simulink model "UDPsimulink"  (R2021a)
settings: Solver=VariableStepAuto  StartTime=0.0  StopTime=inf  RelTol=1e-3
libraries: hostiolib x1, instrumentlib x1
settings Model: EnablePacing=on  Creator=sanja  LastModifiedBy=sanja

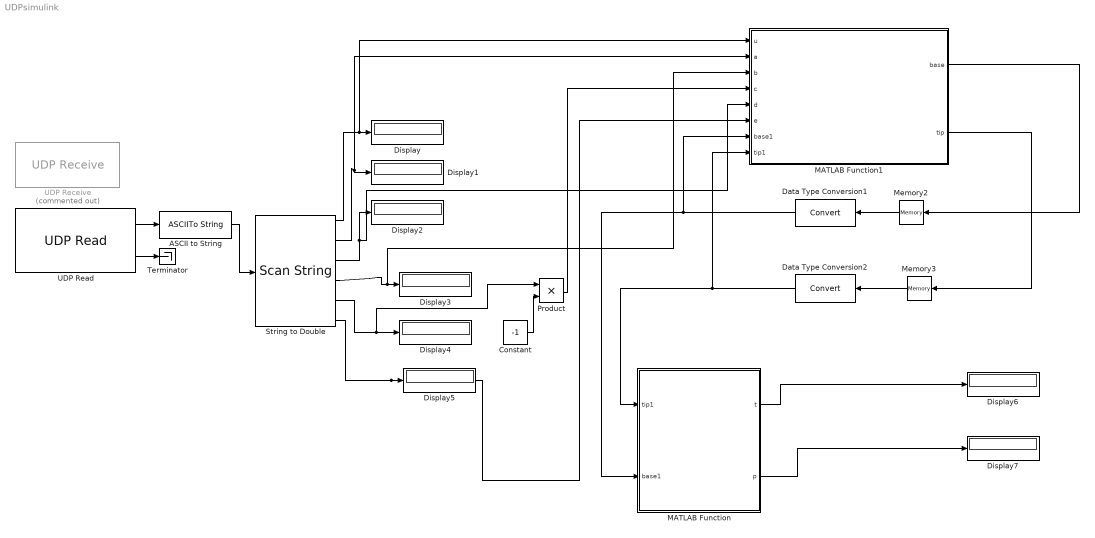
== system UDPsimulink ==
  ASCII to String : ASCIIToString
  Constant : Constant  Value=-1
  Data Type Conversion1 : DataTypeConversion
  Data Type Conversion2 : DataTypeConversion
  Display{,1..7} (8 alike) : Display
  MATLAB Function : MATLAB Function  TreatAsAtomicUnit=on
  MATLAB Function1 : MATLAB Function  TreatAsAtomicUnit=on
  Memory2 : Memory  InitialCondition=[0.0,0,0,0,0,1]  InheritSampleTime=on
  Memory3 : Memory  InitialCondition=[1.0,0,0,0,0,1]  InheritSampleTime=on
  Product : Product
  String to Double : ScanString  Format="\"%f %f %f %f %f %f\""
  Terminator : Terminator
  UDP Read : hostiolib/UDP Read  localURL='0.0.0.0'  localPort=60002  remoteURL='localhost'  remotePort=-1  recvBufferSize=1024  dims=255  signalDatatype=uint8  isVarSize=off  showBlockingTime=on  blockingTime=0  sampletime=0.001  blockPlatform=HOST  hoistedMaskSrc=UDP Read/UDP Read Sim/UDP Read
      settings: SourceProductBaseCode=HW
  UDP Receive : instrumentlib/UDP Receive  Commented=on  Host=localhost  Port=60001  LocalPort=60002  EnablePortSharing=off  GetLatestData=off  DataSize="[1  9]"  DataType=uint8  ASCIIFormatting=%f %f  Terminator=127  ByteOrder=BigEndian  EnableBlockingMode=on  Timeout=10  SampleTime=0.01  LocalAddress=localhost
  wires:
  ASCII to String/1 -> String to Double/1
  String to Double/1 -> MATLAB Function1/1(u), Display/1
  UDP Read/2 -> Terminator/1
  UDP Read/1 -> ASCII to String/1
  String to Double/3 -> MATLAB Function1/5(d), Display2/1
  String to Double/5 -> Product/1, Display4/1
  String to Double/6 -> MATLAB Function1/6(e), Display5/1
  String to Double/2 -> Display1/1, MATLAB Function1/2(a)
  String to Double/4 -> MATLAB Function1/3(b), Display3/1
  MATLAB Function/1(t) -> Display6/1
  MATLAB Function/2(p) -> Display7/1
  Memory2/1 -> Data Type Conversion1/1
  MATLAB Function1/1(base) -> Memory2/1
  Data Type Conversion1/1 -> MATLAB Function/2(base1), MATLAB Function1/7(base1)
  Memory3/1 -> Data Type Conversion2/1
  MATLAB Function1/2(tip) -> Memory3/1
  Data Type Conversion2/1 -> MATLAB Function/1(tip1), MATLAB Function1/8(tip1)
  Constant/1 -> Product/2
  Product/1 -> MATLAB Function1/4(c)

== matlab function UDPsimulink/MATLAB Function1 ==
  data: u input; base output; a input; b input; c input; d input; e input; base1 input; tip1 input; tip output
function [base,tip]= fcn(u,a,b,c,d,e,base1,tip1)
if u==0.0
    %base1=[double(u),double(a),double(b),double(c),double(d),double(e)];
    base1(1)=double(u);
    base1(2)=double(a);
    base1(3)=double(b);
    base1(4)=double(c);
    base1(5)=double(d);
    base1(6)=double(e);
elseif u==1.0
    %tip1=[double(u),double(a),double(b),double(c),double(d),double(e)];
    tip1(1)=double(u);
    tip1(2)=double(a);
    tip1(3)=double(b);
    tip1(4)=double(c);
    tip1(5)=double(d);
    tip1(6)=double(e);
end
    base=base1;
    tip=tip1;

== matlab function UDPsimulink/MATLAB Function ==
  data: tip1 input; t output; base1 input; p output
function [t,p]= fcn(tip1,base1)

base_start=[0,0,0,1];
tip_start=[0,0,0,1];

tip=[tip1(3),tip1(4),tip1(5),tip1(6)];
base=[base1(3),base1(4),base1(5),base1(6)];

tip_relative_base=quatmultiply(quatmultiply(tip,quatinv(tip_start)),quatinv(quatmultiply(base,quatinv(base_start))));

rotMat = quat2tform(tip_relative_base);
phi=acos(rotMat(3,3));

%optimizing
f=@(x)optfun(x,phi);
optAngle=fminsearch(f,0);

rotVal=[optAngle phi];


t= rad2deg(rotVal(1));
p=rad2deg(rotVal(2));


function cost=optfun(ang,phi)

R11=(cos(ang)^2)*cos(phi) + sin(ang)^2;
R12=cos(ang)*sin(ang)*(cos(phi)-1);
R13=cos(ang)*sin(phi);
R22=(sin(ang^2))*cos(phi) + cos(ang)^2;
R23=sin(ang)*sin(phi);
R33=cos(phi);

rotMat_model=[R11 R12 R13 R22 R23 R33];
rotMat_measured=[rotMat(1,1) rotMat(1,2) rotMat(1,3) rotMat(2,2) rotMat(2,3) rotMat(3,3)];
delta=rotMat_model-rotMat_measured;

cost=norm(delta);


end

end
